simulink model "cat_mouse"  (R2018b)
settings: Solver=ode45  StartTime=0.0  StopTime=200  MaxStep=0.006  MinStep=0.0001  RelTol=1e-3  EnableMultiTasking=on
undefined symbols (not defined in the file or in its folder): a, b, c
libraries: simulink x1
settings Model: Creator=Administrator  LastModifiedBy=xiezhh
settings SolverCC: InitialStep=0.005
settings DataIOCC: LimitDataPoints=on  SaveFormat=Array  SignalLoggingSaveFormat=ModelDataLogs
settings OptimizationCC: ExpressionDepthLimit=2147483647  InitFltsAndDblsToZero=on  LifeSpan=inf
settings DebuggingCC: UnderspecifiedInitializationDetection=Classic  MergeDetectMultiDrivingBlocksExec=none  SolverPrmCheckMsg=warning  FcnCallInpInsideContextMsg=warning  AllowSymbolicDim=off  StateNameClashWarn=warning  SFUnexpectedBacktrackingDiag=warning  SFNoUnconditionalDefaultTransitionDiag=warning  SFExecutionAtInitializationDiag=none
settings HardwareCC: ProdBitPerPointer=32  ProdBitPerSizeT=32  ProdBitPerPtrDiffT=32  ProdLargestAtomicFloat=None  ProdIntDivRoundTo=Undefined  ProdEndianess=Unspecified  ProdWordSize=32  ProdHWDeviceType=32-bit Generic
settings ModelReferenceCC: PropagateSignalLabelsOutOfModel=off
settings SFSimCC: SimUseLocalCustomCode=off
settings RTWCC: RTWUseLocalCustomCode=off
settings CodeAppCC: StateflowObjectComments=on
settings GRTTargetCC: TargetLangStandard=C89/C90 (ANSI)  GeneratePreprocessorConditionals=Disable all  CombineOutputUpdateFcns=off  GRTInterface=on
settings ConfigComp: CovMetricSettings=dw  CovHtmlReporting=on  CovSaveCumulativeToWorkspaceVar=on  CovSaveSingleToWorkspaceVar=on  CovExternalEMLEnable=off  CovSFcnEnable=off

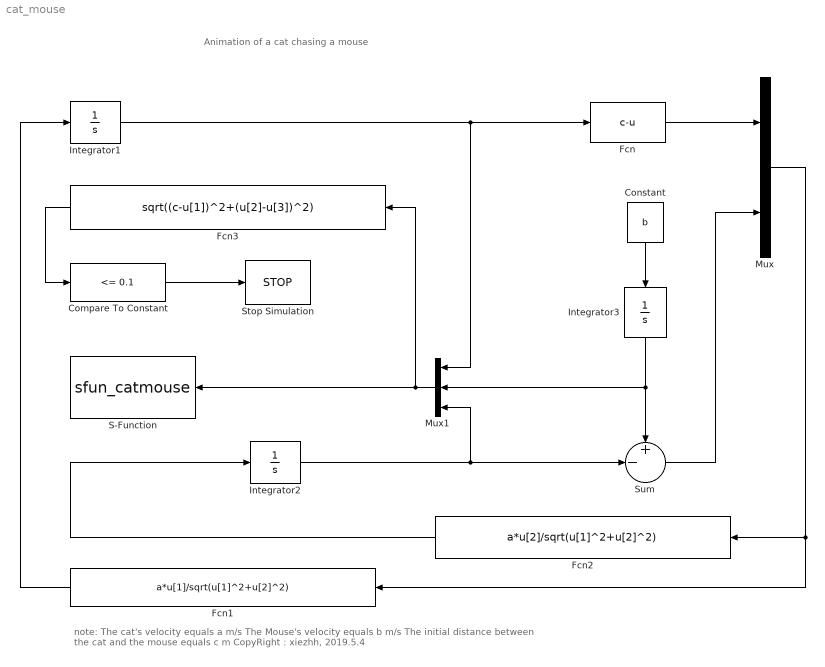
== system cat_mouse ==
  note: Animation of a cat chasing a mouse
  note: note:
      | The cat's velocity equals a m/s
      | The Mouse's velocity equals b m/s
      | The initial distance between the cat and the mouse equals c m
      | CopyRight : xiezhh, 2019.5.4
  Compare To Constant : simulink/Logic and Bit Operations/Compare To Constant  relop=<=  const=0.1  OutDataTypeStr=boolean  ZeroCross=off
  Constant : Constant  Value=b
  Fcn : Fcn  Expr=c-u
  Fcn1 : Fcn  Expr=a*u[1]/sqrt(u[1]^2+u[2]^2)
  Fcn2 : Fcn  Expr=a*u[2]/sqrt(u[1]^2+u[2]^2)
  Fcn3 : Fcn  Expr=sqrt((c-u[1])^2+(u[2]-u[3])^2)
  Integrator1 : Integrator
  Integrator2 : Integrator
  Integrator3 : Integrator
  Mux : Mux  Inputs=2
  Mux1 : Mux  Inputs=3
  S-Function : S-Function  FunctionName=sfun_catmouse  Parameters=12,6,20  SFunctionDeploymentMode=off  EnableBusSupport=off
      mask Display: image(imread('catandmouse.jpg'));
  Stop Simulation : Stop
  Sum : Sum  Inputs=+-|
  wires:
  Mux/1 -> Fcn2/1, Fcn1/1
  Fcn2/1 -> Integrator2/1
  Fcn1/1 -> Integrator1/1
  Integrator1/1 -> Fcn/1, Mux1/1
  Fcn/1 -> Mux/1
  Sum/1 -> Mux/2
  Mux1/1 -> S-Function/1, Fcn3/1
  Integrator2/1 -> Sum/2, Mux1/3
  Integrator3/1 -> Sum/1, Mux1/2
  Constant/1 -> Integrator3/1
  Fcn3/1 -> Compare To Constant/1
  Compare To Constant/1 -> Stop Simulation/1
